simulink model "WaterRunner_closed2"  (R2013a)
settings: Solver=ode23s  StartTime=0.0  StopTime=10  RelTol=1e-3
values from neighbouring files (symbols this model uses):
  Ac = [sum(Ay), sum(Ath), sum(Aph) ... (first row only)    [SimParam_hopper.m]    (also in simParam.m = [2*sum(Ay), 2*sum(Ath))
  dTorqueAmp = 1e-2    (= 0.01)    [SimParam_hopper.m]
  dTorqueFreq = 0.5    [SimParam_hopper.m]    (also in simParam.m = 3.14159265359)
  Filter_Coef = 1000    [SimParam_hopper.m]    (also in simParam.m)
  freq = findSSinput(y,b_water,k_water,A,Fratio,mass*g/4,w0)    [SimParam_hopper.m]    (also in findParams.m = freqs(k); simParam.m; sweepDFomega.m = FREQ(k))
  Gc = [sum(G) - mass*g ; Lx'*G ; Lz'*G]    [SimParam_hopper.m]    (also in simParam.m = [2*sum(G) - mass*g ; Lx'*G ])
  Kdf = 0.25    [SimParam_hopper.m]    (also in simParam.m = 0)
  Ke = diag([0 1])    [simParam.m]
  Mc = [mass 0 0; 0 Ix 0 ; 0 0 Iz]    [SimParam_hopper.m]    (also in simParam.m = [mass 0 ; 0 Ix])
  nullProj = eye(8) - pinvBc*Bc    [SimParam_hopper.m]    (also in simParam.m = eye(4) - pinvBc*Bc)
  omega_0 = freq*ones(8,1)    [SimParam_hopper.m]    (also in findParams.m = freq*ones(4,1); simParam.m = freq*ones(4,1); sweepDFomega.m = freq*ones(4,1))
  pinvBc = pinv(Bc)    [SimParam_hopper.m]    (also in simParam.m)
  tail_density = CF_density    (= 1790)    [simParam.m]
  tail_length = 0.1    [simParam.m]
  theta = 0 *pi/180    (= 0)    [SimParam_hopper.m]    (also in simParam.m)
  y = 0.02    [SimParam_hopper.m]    (also in simParam.m = 0.015)
undefined symbols (not defined in the file or in its folder): X, Y, Z
undefined symbols (not defined in the file): cw_FL_HL, cw_FR_FL, cw_FR_HR, cw_HR_HL, FL_HL_lag, FR_FL_lag, FR_HR_lag, HR_HL_lag, K_d, K_i, K_p, phi0, tail_pad_radius, theta0, water_level, y0
libraries: nesl_utility x38, sm_lib x35, WaterRunner_lib_2 x11, dspstat3 x4, simulink x2
(part 2 of 4)

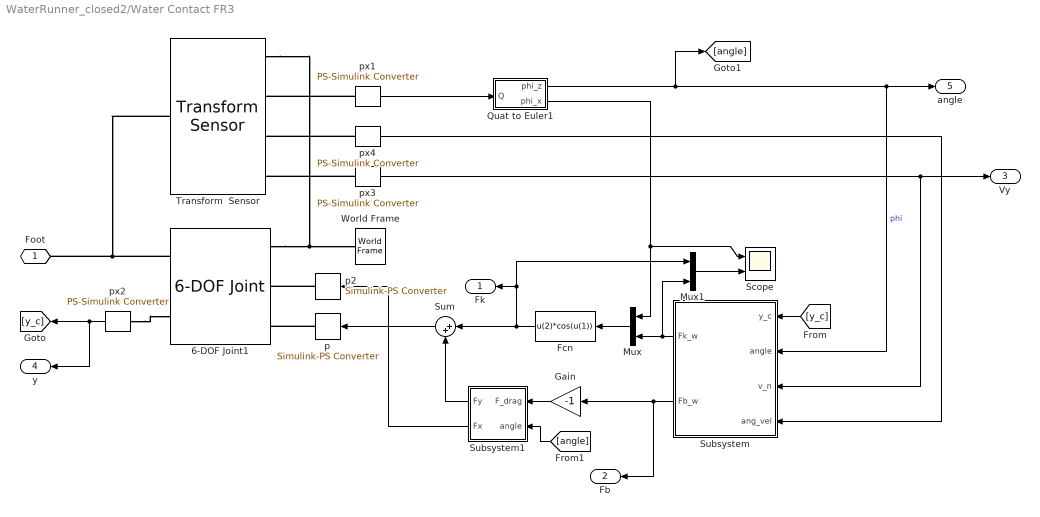
== system WaterRunner_closed2/Water Contact FR3 ==
  6-DOF Joint1 : sm_lib/Joints/6-DOF Joint  SenseConstraintForceX=off  SenseConstraintForceY=off  SenseConstraintForceZ=off  SenseConstraintTorqueX=off  SenseConstraintTorqueY=off  SenseConstraintTorqueZ=off  ConstraintWrenchDir=FollowerOnBase  ConstraintWrenchFrame=BaseFrame  PxEquilibriumPosition=0  PxEquilibriumPositionUnits=m  PxSpringStiffness=0  PxSpringStiffnessUnits=N/m  PxDampingCoefficient=0  PxDampingCoefficientUnits=N/(m/s)  PxActuationMode=TorqueForceActuation  PxSensePosition=off  PxSenseVelocity=off  PxSenseAcceleration=off  PxSenseTorqueForce=off  PxPositionTargetValue=0  PxPositionTargetValueUnits=m  PxPositionTargetSpecify=off  PxPositionTargetPriority=High  PxVelocityTargetValue=0  PxVelocityTargetValueUnits=m/s  PxVelocityTargetSpecify=off  PxVelocityTargetPriority=High  PyEquilibriumPosition=0  PyEquilibriumPositionUnits=m  PySpringStiffness=0  PySpringStiffnessUnits=N/m  PyDampingCoefficient=0  PyDampingCoefficientUnits=N/(m/s)  PyActuationMode=TorqueForceActuation  PySensePosition=on  PySenseVelocity=off  PySenseAcceleration=off  PySenseTorqueForce=off  PyPositionTargetValue=0  PyPositionTargetValueUnits=m  PyPositionTargetSpecify=off  PyPositionTargetPriority=High  PyVelocityTargetValue=0  PyVelocityTargetValueUnits=m/s  PyVelocityTargetSpecify=off  PyVelocityTargetPriority=High  PzEquilibriumPosition=0  PzEquilibriumPositionUnits=m  PzSpringStiffness=0  PzSpringStiffnessUnits=N/m  PzDampingCoefficient=0  PzDampingCoefficientUnits=N/(m/s)  PzActuationMode=NoActuation  PzSensePosition=off  PzSenseVelocity=off  PzSenseAcceleration=off  PzSenseTorqueForce=off  PzPositionTargetValue=0  PzPositionTargetValueUnits=m  PzPositionTargetSpecify=off  PzPositionTargetPriority=High  PzVelocityTargetValue=0  PzVelocityTargetValueUnits=m/s  PzVelocityTargetSpecify=off  PzVelocityTargetPriority=High  SphDefPosRotationMethod=None  SphDefPosRotationAngleUnits=deg  SphDefPosRotationStandardAxis=+Z  SphDefPosRotationAngle=0  SphDefPosRotationArbitraryAxis=[0 0 1]  SphDefPosFollAlignAxisA=+X  SphDefPosBaseAlignAxisA=+Y  SphDefPosFollAlignAxisB=+Y  SphDefPosBaseAlignAxisB=+Z  SphEqPosRotationMethod=None  SphEqPosRotationAngleUnits=deg  SphEqPosRotationStandardAxis=+Z  SphEqPosRotationAngle=0  SphEqPosRotationArbitraryAxis=[0 0 1]  SphEqPosFollAlignAxisA=+X  SphEqPosBaseAlignAxisA=+Y  SphEqPosFollAlignAxisB=+Y  SphEqPosBaseAlignAxisB=+Z  SphSpringStiffness=0  SphSpringStiffnessUnits=N*m/deg  SphDampingCoefficient=0  SphDampingCoefficientUnits=N*m/(deg/s)  SphActuateTorqueX=off  SphActuateTorqueY=off  SphActuateTorqueZ=off  SphActuateTorque=off  SphActuationMode=NoActuation  SphActuationFrame=BaseFrame  SphSensePosition=off  SphSenseVelocityX=off  SphSenseVelocityY=off  SphSenseVelocityZ=off  SphSenseVelocity=off  SphSenseAccelerationX=off  SphSenseAccelerationY=off  SphSenseAccelerationZ=off  SphSenseAcceleration=off  SphSenseTorqueX=off  SphSenseTorqueY=off  SphSenseTorqueZ=off  SphSenseTorqueForce=off  SphSensingFrame=BaseFrame  SphPositionTargetRotationMethod=None  SphPositionTargetRotationAngleUnits=deg  SphPositionTargetRotationStandardAxis=+Z  SphPositionTargetRotationAngle=0  SphPositionTargetRotationArbitraryAxis=[0 0 1]  SphPositionTargetFollAlignAxisA=+X  SphPositionTargetBaseAlignAxisA=+Y  SphPositionTargetFollAlignAxisB=+Y  SphPositionTargetBaseAlignAxisB=+Z  SphPositionTargetSpecify=off  SphPositionTargetPriority=High  SphVelocityTargetValue=[0 0 0]  SphVelocityTargetValueUnits=deg/s  SphVelocityTargetSpecify=off  SphVelocityTargetPriority=High  SphVelocityTargetInFollowerFrame=on  BlockFunction=simmechanics.library.joints.sixdof_joint
  Fcn : Fcn  Expr=u(2)*cos(u(1))
  Gain : Gain  Gain=-1
  Mux : Mux  Inputs=2
  Mux1 : Mux  Inputs=2
  Quat to Euler1 : Subsystem
  Scope : Scope  NumInputPorts=2
      settings: YMin=-0.19~0  YMax=0.04~0.7  SaveName=ScopeData3
  Subsystem : Subsystem
  Subsystem1 : Subsystem
  Sum : Sum  Inputs=|++
  Transform  Sensor : sm_lib/Frames and  Transforms/Transform  Sensor  MeasurementFrame=NonRotatingBase  SenseAngle=off  SenseAxis=off  SenseAngle1=off  SenseAngle2=off  SenseAngle3=off  SenseQ=on  SenseR=off  SenseOmegaX=off  SenseOmegaY=off  SenseOmegaZ=on  SenseOmega1=off  SenseOmega2=off  SenseOmega3=off  SenseQDot=off  SenseRDot=off  SenseAlphaX=off  SenseAlphaY=off  SenseAlphaZ=off  SenseAlpha1=off  SenseAlpha2=off  SenseAlpha3=off  SenseQDDot=off  SenseRDDot=off  SenseX=off  SenseY=off  SenseZ=off  SenseRad=off  SenseAzim=off  SenseDist=off  SenseInc=off  SenseXDot=off  SenseYDot=on  SenseZDot=off  SenseRadDot=off  SenseAzimDot=off  SenseDistDot=off  SenseIncDot=off  SenseXDDot=off  SenseYDDot=off  SenseZDDot=off  SenseRadDDot=off  SenseAzimDDot=off  SenseDistDDot=off  SenseIncDDot=off  BlockFunction=simmechanics.library.frames_transforms.transform_sensor
  World Frame : sm_lib/Frames and  Transforms/World Frame  BlockFunction=simmechanics.library.frames_transforms.world_frame
  p : nesl_utility/Simulink-PS Converter  PhysicalDomain=network_engine_domain  SubClassName=ps_input  LeftPortType=input  RightPortType=output  PseudoPeriodic=off  Frequencies=[]  NoiseDistribution=none  NoiseParameters=[]  Unit=1  AffineConversion=off  InputFiltering=off  SimscapeFilterOrder=1  InputFilterTimeConstant=.001  UdotUserProvided=[]
  p2 : nesl_utility/Simulink-PS Converter  PhysicalDomain=network_engine_domain  SubClassName=ps_input  LeftPortType=input  RightPortType=output  PseudoPeriodic=off  Frequencies=[]  NoiseDistribution=none  NoiseParameters=[]  Unit=1  AffineConversion=off  InputFiltering=off  SimscapeFilterOrder=1  InputFilterTimeConstant=.001  UdotUserProvided=[]
  px{1..4} (4 alike) : nesl_utility/PS-Simulink Converter  PhysicalDomain=network_engine_domain  SubClassName=ps_output  LeftPortType=input  RightPortType=output  PseudoPeriodic=off  Frequencies=[]  Unit=1  AffineConversion=off
  Foot : PMIOPort  Port=1  Side=Left
  Fk : Outport
  Fb : Outport  Port=2
  Vy : Outport  Port=3
  y : Outport  Port=4
  angle : Outport  Port=5
  wires:
  Subsystem/2(Fb_w) -> Gain/1, Fb/1
  px3/1 -> Vy/1, Subsystem/3(v_n)
  Quat to Euler1/1(phi_z) -> [angle], Subsystem/2(angle), angle/1  "phi"
  px1/1 -> Quat to Euler1/1(Q)
  px4/1 -> Subsystem/4(ang_vel)
  px2/1 -> [y_c], y/1
  [y_c] -> Subsystem/1(y_c)
  [angle] -> Subsystem1/2(angle)
  Sum/1 -> p/1
  Subsystem1/1(Fy) -> Sum/2
  Gain/1 -> Subsystem1/1(F_drag)
  Subsystem1/2(Fx) -> p2/1
  Subsystem/1(Fk_w) -> Mux1/2, Mux/2
  Mux/1 -> Fcn/1
  Fcn/1 -> Mux1/1, Fk/1, Sum/1
  Quat to Euler1/2(phi_x) -> Mux/1, Scope/1
  Mux1/1 -> Scope/2
  connections:
  Transform  Sensor/RConn1 -- World Frame/RConn1 -- 6-DOF Joint1/LConn1
  Transform  Sensor/LConn1 -- Foot/RConn1 -- 6-DOF Joint1/RConn1
  px2/LConn1 -- 6-DOF Joint1/RConn2
  p/RConn1 -- 6-DOF Joint1/LConn3
  px1/LConn1 -- Transform  Sensor/RConn2
  p2/RConn1 -- 6-DOF Joint1/LConn2
  px3/LConn1 -- Transform  Sensor/RConn4
  px4/LConn1 -- Transform  Sensor/RConn3

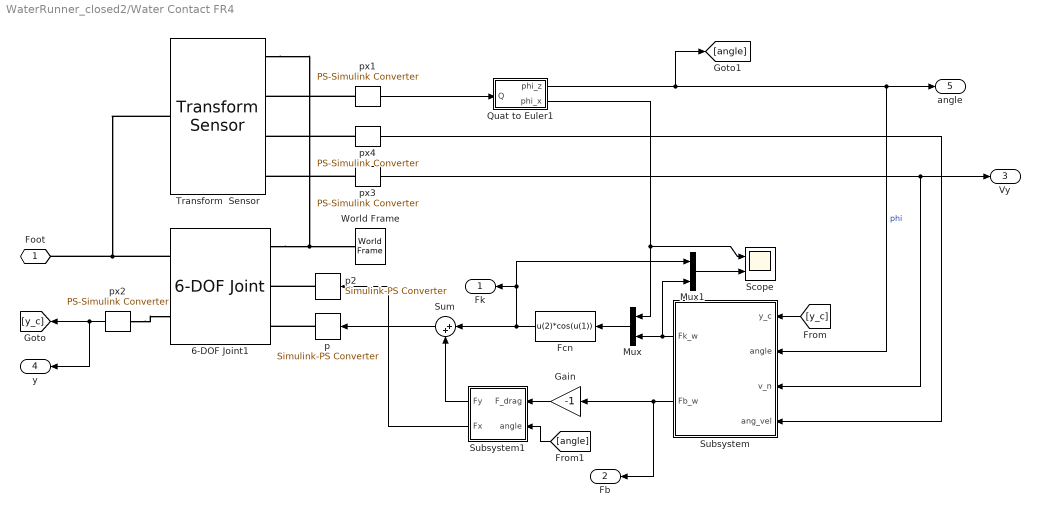
== system WaterRunner_closed2/Water Contact FR4 ==
  6-DOF Joint1 : sm_lib/Joints/6-DOF Joint  SenseConstraintForceX=off  SenseConstraintForceY=off  SenseConstraintForceZ=off  SenseConstraintTorqueX=off  SenseConstraintTorqueY=off  SenseConstraintTorqueZ=off  ConstraintWrenchDir=FollowerOnBase  ConstraintWrenchFrame=BaseFrame  PxEquilibriumPosition=0  PxEquilibriumPositionUnits=m  PxSpringStiffness=0  PxSpringStiffnessUnits=N/m  PxDampingCoefficient=0  PxDampingCoefficientUnits=N/(m/s)  PxActuationMode=TorqueForceActuation  PxSensePosition=off  PxSenseVelocity=off  PxSenseAcceleration=off  PxSenseTorqueForce=off  PxPositionTargetValue=0  PxPositionTargetValueUnits=m  PxPositionTargetSpecify=off  PxPositionTargetPriority=High  PxVelocityTargetValue=0  PxVelocityTargetValueUnits=m/s  PxVelocityTargetSpecify=off  PxVelocityTargetPriority=High  PyEquilibriumPosition=0  PyEquilibriumPositionUnits=m  PySpringStiffness=0  PySpringStiffnessUnits=N/m  PyDampingCoefficient=0  PyDampingCoefficientUnits=N/(m/s)  PyActuationMode=TorqueForceActuation  PySensePosition=on  PySenseVelocity=off  PySenseAcceleration=off  PySenseTorqueForce=off  PyPositionTargetValue=0  PyPositionTargetValueUnits=m  PyPositionTargetSpecify=off  PyPositionTargetPriority=High  PyVelocityTargetValue=0  PyVelocityTargetValueUnits=m/s  PyVelocityTargetSpecify=off  PyVelocityTargetPriority=High  PzEquilibriumPosition=0  PzEquilibriumPositionUnits=m  PzSpringStiffness=0  PzSpringStiffnessUnits=N/m  PzDampingCoefficient=0  PzDampingCoefficientUnits=N/(m/s)  PzActuationMode=NoActuation  PzSensePosition=off  PzSenseVelocity=off  PzSenseAcceleration=off  PzSenseTorqueForce=off  PzPositionTargetValue=0  PzPositionTargetValueUnits=m  PzPositionTargetSpecify=off  PzPositionTargetPriority=High  PzVelocityTargetValue=0  PzVelocityTargetValueUnits=m/s  PzVelocityTargetSpecify=off  PzVelocityTargetPriority=High  SphDefPosRotationMethod=None  SphDefPosRotationAngleUnits=deg  SphDefPosRotationStandardAxis=+Z  SphDefPosRotationAngle=0  SphDefPosRotationArbitraryAxis=[0 0 1]  SphDefPosFollAlignAxisA=+X  SphDefPosBaseAlignAxisA=+Y  SphDefPosFollAlignAxisB=+Y  SphDefPosBaseAlignAxisB=+Z  SphEqPosRotationMethod=None  SphEqPosRotationAngleUnits=deg  SphEqPosRotationStandardAxis=+Z  SphEqPosRotationAngle=0  SphEqPosRotationArbitraryAxis=[0 0 1]  SphEqPosFollAlignAxisA=+X  SphEqPosBaseAlignAxisA=+Y  SphEqPosFollAlignAxisB=+Y  SphEqPosBaseAlignAxisB=+Z  SphSpringStiffness=0  SphSpringStiffnessUnits=N*m/deg  SphDampingCoefficient=0  SphDampingCoefficientUnits=N*m/(deg/s)  SphActuateTorqueX=off  SphActuateTorqueY=off  SphActuateTorqueZ=off  SphActuateTorque=off  SphActuationMode=NoActuation  SphActuationFrame=BaseFrame  SphSensePosition=off  SphSenseVelocityX=off  SphSenseVelocityY=off  SphSenseVelocityZ=off  SphSenseVelocity=off  SphSenseAccelerationX=off  SphSenseAccelerationY=off  SphSenseAccelerationZ=off  SphSenseAcceleration=off  SphSenseTorqueX=off  SphSenseTorqueY=off  SphSenseTorqueZ=off  SphSenseTorqueForce=off  SphSensingFrame=BaseFrame  SphPositionTargetRotationMethod=None  SphPositionTargetRotationAngleUnits=deg  SphPositionTargetRotationStandardAxis=+Z  SphPositionTargetRotationAngle=0  SphPositionTargetRotationArbitraryAxis=[0 0 1]  SphPositionTargetFollAlignAxisA=+X  SphPositionTargetBaseAlignAxisA=+Y  SphPositionTargetFollAlignAxisB=+Y  SphPositionTargetBaseAlignAxisB=+Z  SphPositionTargetSpecify=off  SphPositionTargetPriority=High  SphVelocityTargetValue=[0 0 0]  SphVelocityTargetValueUnits=deg/s  SphVelocityTargetSpecify=off  SphVelocityTargetPriority=High  SphVelocityTargetInFollowerFrame=on  BlockFunction=simmechanics.library.joints.sixdof_joint
  Fcn : Fcn  Expr=u(2)*cos(u(1))
  Gain : Gain  Gain=-1
  Mux : Mux  Inputs=2
  Mux1 : Mux  Inputs=2
  Quat to Euler1 : Subsystem
  Scope : Scope  NumInputPorts=2
      settings: YMin=-0.19~0  YMax=0.04~0.7  SaveName=ScopeData3
  Subsystem : Subsystem
  Subsystem1 : Subsystem
  Sum : Sum  Inputs=|++
  Transform  Sensor : sm_lib/Frames and  Transforms/Transform  Sensor  MeasurementFrame=NonRotatingBase  SenseAngle=off  SenseAxis=off  SenseAngle1=off  SenseAngle2=off  SenseAngle3=off  SenseQ=on  SenseR=off  SenseOmegaX=off  SenseOmegaY=off  SenseOmegaZ=on  SenseOmega1=off  SenseOmega2=off  SenseOmega3=off  SenseQDot=off  SenseRDot=off  SenseAlphaX=off  SenseAlphaY=off  SenseAlphaZ=off  SenseAlpha1=off  SenseAlpha2=off  SenseAlpha3=off  SenseQDDot=off  SenseRDDot=off  SenseX=off  SenseY=off  SenseZ=off  SenseRad=off  SenseAzim=off  SenseDist=off  SenseInc=off  SenseXDot=off  SenseYDot=on  SenseZDot=off  SenseRadDot=off  SenseAzimDot=off  SenseDistDot=off  SenseIncDot=off  SenseXDDot=off  SenseYDDot=off  SenseZDDot=off  SenseRadDDot=off  SenseAzimDDot=off  SenseDistDDot=off  SenseIncDDot=off  BlockFunction=simmechanics.library.frames_transforms.transform_sensor
  World Frame : sm_lib/Frames and  Transforms/World Frame  BlockFunction=simmechanics.library.frames_transforms.world_frame
  p : nesl_utility/Simulink-PS Converter  PhysicalDomain=network_engine_domain  SubClassName=ps_input  LeftPortType=input  RightPortType=output  PseudoPeriodic=off  Frequencies=[]  NoiseDistribution=none  NoiseParameters=[]  Unit=1  AffineConversion=off  InputFiltering=off  SimscapeFilterOrder=1  InputFilterTimeConstant=.001  UdotUserProvided=[]
  p2 : nesl_utility/Simulink-PS Converter  PhysicalDomain=network_engine_domain  SubClassName=ps_input  LeftPortType=input  RightPortType=output  PseudoPeriodic=off  Frequencies=[]  NoiseDistribution=none  NoiseParameters=[]  Unit=1  AffineConversion=off  InputFiltering=off  SimscapeFilterOrder=1  InputFilterTimeConstant=.001  UdotUserProvided=[]
  px{1..4} (4 alike) : nesl_utility/PS-Simulink Converter  PhysicalDomain=network_engine_domain  SubClassName=ps_output  LeftPortType=input  RightPortType=output  PseudoPeriodic=off  Frequencies=[]  Unit=1  AffineConversion=off
  Foot : PMIOPort  Port=1  Side=Left
  Fk : Outport
  Fb : Outport  Port=2
  Vy : Outport  Port=3
  y : Outport  Port=4
  angle : Outport  Port=5
  wires:
  Subsystem/2(Fb_w) -> Gain/1, Fb/1
  px3/1 -> Vy/1, Subsystem/3(v_n)
  Quat to Euler1/1(phi_z) -> [angle], Subsystem/2(angle), angle/1  "phi"
  px1/1 -> Quat to Euler1/1(Q)
  px4/1 -> Subsystem/4(ang_vel)
  px2/1 -> [y_c], y/1
  [y_c] -> Subsystem/1(y_c)
  [angle] -> Subsystem1/2(angle)
  Sum/1 -> p/1
  Subsystem1/1(Fy) -> Sum/2
  Gain/1 -> Subsystem1/1(F_drag)
  Subsystem1/2(Fx) -> p2/1
  Subsystem/1(Fk_w) -> Mux1/2, Mux/2
  Mux/1 -> Fcn/1
  Fcn/1 -> Mux1/1, Fk/1, Sum/1
  Quat to Euler1/2(phi_x) -> Mux/1, Scope/1
  Mux1/1 -> Scope/2
  connections:
  Transform  Sensor/RConn1 -- World Frame/RConn1 -- 6-DOF Joint1/LConn1
  Transform  Sensor/LConn1 -- Foot/RConn1 -- 6-DOF Joint1/RConn1
  px2/LConn1 -- 6-DOF Joint1/RConn2
  p/RConn1 -- 6-DOF Joint1/LConn3
  px1/LConn1 -- Transform  Sensor/RConn2
  p2/RConn1 -- 6-DOF Joint1/LConn2
  px3/LConn1 -- Transform  Sensor/RConn4
  px4/LConn1 -- Transform  Sensor/RConn3

== system WaterRunner_closed2/desired output ==
  Mux1 : Mux  Inputs=2
  m : Constant  Value=y
  m1 : Constant  Value=theta
  desired output : Outport
  wires:
  m/1 -> Mux1/1  "height"
  Mux1/1 -> desired output/1
  m1/1 -> Mux1/2

== system WaterRunner_closed2/observer ==
  Gain : Gain  Gain=-1
  Gain1 : Gain  Gain=-1
  Integrator : Integrator
  Integrator1 : Integrator
  Mux{,1..2,5} (4 alike) : Mux  Inputs=2
  PS-Simulink Converter{,1..5} (6 alike) : nesl_utility/PS-Simulink Converter  PhysicalDomain=network_engine_domain  SubClassName=ps_output  LeftPortType=input  RightPortType=output  PseudoPeriodic=off  Frequencies=[]  Unit=1  AffineConversion=off
  Transform  Sensor : sm_lib/Frames and  Transforms/Transform  Sensor  MeasurementFrame=World  SenseAngle=off  SenseAxis=off  SenseAngle1=off  SenseAngle2=off  SenseAngle3=off  SenseQ=off  SenseR=off  SenseOmegaX=on  SenseOmegaY=off  SenseOmegaZ=on  SenseOmega1=off  SenseOmega2=off  SenseOmega3=off  SenseQDot=off  SenseRDot=off  SenseAlphaX=on  SenseAlphaY=off  SenseAlphaZ=on  SenseAlpha1=off  SenseAlpha2=off  SenseAlpha3=off  SenseQDDot=off  SenseRDDot=off  SenseX=off  SenseY=on  SenseZ=off  SenseRad=off  SenseAzim=off  SenseDist=off  SenseInc=off  SenseXDot=off  SenseYDot=off  SenseZDot=off  SenseRadDot=off  SenseAzimDot=off  SenseDistDot=off  SenseIncDot=off  SenseXDDot=off  SenseYDDot=on  SenseZDDot=off  SenseRadDDot=off  SenseAzimDDot=off  SenseDistDDot=off  SenseIncDDot=off  BlockFunction=simmechanics.library.frames_transforms.transform_sensor
  averaging1 : Subsystem  mask{T_win=2*pi/freq, x_init=y0}
      mask prompts: T_win "window (s)"; x_init "Initial condition"
  averaging2 : Subsystem  mask{T_win=2*pi/freq, x_init=0}
      mask prompts: T_win "window (s)"; x_init "Initial condition"
  averaging3 : Subsystem  mask{T_win=2*pi/freq, x_init=[0 0]}
      mask prompts: T_win "window (s)"; x_init "Initial condition"
  averaging5 : Subsystem  mask{T_win=2*pi/freq, x_init=[theta0 phi0]}
      mask prompts: T_win "window (s)"; x_init "Initial condition"
  Base : PMIOPort  Port=1  Side=Left
  Follower : PMIOPort  Port=2  Side=Left
  output : Outport
  accel : Outport  Port=2
  wires:
  Mux5/1 -> output/1
  Mux/1 -> averaging5/1(in)
  PS-Simulink Converter/1 -> Integrator/1
  Integrator1/1 -> Mux/2
  Integrator/1 -> Gain/1
  PS-Simulink Converter1/1 -> Integrator1/1
  PS-Simulink Converter2/1 -> averaging1/1(in)
  averaging1/1(out) -> Mux5/1
  Mux2/1 -> accel/1
  Mux1/1 -> averaging3/1(in)
  PS-Simulink Converter4/1 -> Mux1/2
  PS-Simulink Converter3/1 -> Gain1/1
  PS-Simulink Converter5/1 -> averaging2/1(in)
  averaging2/1(out) -> Mux2/1
  averaging5/1(out) -> Mux5/2
  averaging3/1(out) -> Mux2/2
  Gain/1 -> Mux/1
  Gain1/1 -> Mux1/1
  connections:
  Transform  Sensor/LConn1 -- Base/RConn1
  PS-Simulink Converter/LConn1 -- Transform  Sensor/RConn2
  Follower/RConn1 -- Transform  Sensor/RConn1
  PS-Simulink Converter1/LConn1 -- Transform  Sensor/RConn3
  PS-Simulink Converter2/LConn1 -- Transform  Sensor/RConn6
  PS-Simulink Converter3/LConn1 -- Transform  Sensor/RConn4
  PS-Simulink Converter4/LConn1 -- Transform  Sensor/RConn5
  PS-Simulink Converter5/LConn1 -- Transform  Sensor/RConn7

== system WaterRunner_closed2/CPG_Network/FL_HL lag ==
  In1 : Inport
  In2 : Inport  Port=2
  Constant : Constant  Value=d_phase
  Gain : Gain  Gain=-1
  Sum : Sum  Inputs=--+
  sin : Fcn  Expr=coupling_weight*sin(u(1))
  Out1 : Outport
  Out2 : Outport  Port=2
  wires:
  Sum/1 -> sin/1
  sin/1 -> Gain/1, Out1/1
  Constant/1 -> Sum/2
  In1/1 -> Sum/1
  In2/1 -> Sum/3
  Gain/1 -> Out2/1

== system WaterRunner_closed2/CPG_Network/FR_FL lag ==
  In1 : Inport
  In2 : Inport  Port=2
  Constant : Constant  Value=d_phase
  Gain : Gain  Gain=-1
  Sum : Sum  Inputs=--+
  sin : Fcn  Expr=coupling_weight*sin(u(1))
  Out1 : Outport
  Out2 : Outport  Port=2
  wires:
  Sum/1 -> sin/1
  sin/1 -> Gain/1, Out1/1
  Constant/1 -> Sum/2
  In1/1 -> Sum/1
  In2/1 -> Sum/3
  Gain/1 -> Out2/1

== system WaterRunner_closed2/CPG_Network/FR_HR lag ==
  In1 : Inport
  In2 : Inport  Port=2
  Constant : Constant  Value=d_phase
  Gain : Gain  Gain=-1
  Sum : Sum  Inputs=--+
  sin : Fcn  Expr=coupling_weight*sin(u(1))
  Out1 : Outport
  Out2 : Outport  Port=2
  wires:
  Gain/1 -> Out2/1
  In2/1 -> Sum/3
  In1/1 -> Sum/1
  Constant/1 -> Sum/2
  sin/1 -> Out1/1, Gain/1
  Sum/1 -> sin/1

== system WaterRunner_closed2/CPG_Network/Front_Left ==
  force : Inport
  Constant3 : Constant  Value=freq
  Integrator3 : Integrator  InitialCondition=init_phi + 0.001*rand
  Mod 2pi : Fcn  Expr=atan2(sin(u(1)-pi),cos(u(1)-pi))+pi
  Sum2 : Sum  Inputs=|++
  vel : Outport
  phase : Outport  Port=2
  wires:
  force/1 -> Sum2/2
  Sum2/1 -> vel/1, Integrator3/1
  Constant3/1 -> Sum2/1
  Integrator3/1 -> Mod 2pi/1
  Mod 2pi/1 -> phase/1

== system WaterRunner_closed2/CPG_Network/Front_Right ==
  force : Inport
  Constant3 : Constant  Value=freq
  Integrator3 : Integrator  InitialCondition=init_phi + 0.001*rand
  Mod 2pi : Fcn  Expr=atan2(sin(u(1)-pi),cos(u(1)-pi))+pi
  Sum2 : Sum  Inputs=|++
  vel : Outport
  phase : Outport  Port=2
  wires:
  Mod 2pi/1 -> phase/1
  Integrator3/1 -> Mod 2pi/1
  Constant3/1 -> Sum2/1
  Sum2/1 -> Integrator3/1, vel/1
  force/1 -> Sum2/2

== system WaterRunner_closed2/CPG_Network/HR_HL lag ==
  In1 : Inport
  In2 : Inport  Port=2
  Constant : Constant  Value=d_phase
  Gain : Gain  Gain=-1
  Sum : Sum  Inputs=--+
  sin : Fcn  Expr=coupling_weight*sin(u(1))
  Out1 : Outport
  Out2 : Outport  Port=2
  wires:
  Gain/1 -> Out2/1
  In2/1 -> Sum/3
  In1/1 -> Sum/1
  Constant/1 -> Sum/2
  sin/1 -> Out1/1, Gain/1
  Sum/1 -> sin/1

== system WaterRunner_closed2/CPG_Network/Hind_Left ==
  force : Inport
  Constant3 : Constant  Value=freq
  Integrator3 : Integrator  InitialCondition=init_phi + 0.001*rand
  Mod 2pi : Fcn  Expr=atan2(sin(u(1)-pi),cos(u(1)-pi))+pi
  Sum2 : Sum  Inputs=|++
  vel : Outport
  phase : Outport  Port=2
  wires:
  force/1 -> Sum2/2
  Sum2/1 -> vel/1, Integrator3/1
  Constant3/1 -> Sum2/1
  Integrator3/1 -> Mod 2pi/1
  Mod 2pi/1 -> phase/1

== system WaterRunner_closed2/CPG_Network/Hind_Right ==
  force : Inport
  Constant3 : Constant  Value=freq
  Integrator3 : Integrator  InitialCondition=init_phi + 0.001*rand
  Mod 2pi : Fcn  Expr=atan2(sin(u(1)-pi),cos(u(1)-pi))+pi
  Sum2 : Sum  Inputs=|++
  vel : Outport
  phase : Outport  Port=2
  wires:
  force/1 -> Sum2/2
  Sum2/1 -> vel/1, Integrator3/1
  Constant3/1 -> Sum2/1
  Integrator3/1 -> Mod 2pi/1
  Mod 2pi/1 -> phase/1

== system WaterRunner_closed2/CPG_Network/split FL ==
  w_pos : Inport
  phase : Inport  Port=2
  w_neg : Inport  Port=3
  Product : Product  RndMeth=Zero
  Product1 : Product  RndMeth=Zero
  Sum2 : Sum  Inputs=|++
  enable : Subsystem
  Force : Outport
  wires:
  Product/1 -> Sum2/1
  w_pos/1 -> Product/1
  w_neg/1 -> Product1/1
  Product1/1 -> Sum2/2
  enable/1(pos) -> Product/2
  enable/2(neg) -> Product1/2
  Sum2/1 -> Force/1
  phase/1 -> enable/1(in)

== system WaterRunner_closed2/CPG_Network/split FL1 ==
  w_pos : Inport
  phase : Inport  Port=2
  w_neg : Inport  Port=3
  Product : Product  RndMeth=Zero
  Product1 : Product  RndMeth=Zero
  Sum2 : Sum  Inputs=|++
  enable : Subsystem
  Force : Outport
  wires:
  Product/1 -> Sum2/1
  w_pos/1 -> Product/1
  w_neg/1 -> Product1/1
  Product1/1 -> Sum2/2
  enable/1(pos) -> Product/2
  enable/2(neg) -> Product1/2
  Sum2/1 -> Force/1
  phase/1 -> enable/1(in)

== system WaterRunner_closed2/CPG_Network/split FL2 ==
  w_pos : Inport
  phase : Inport  Port=2
  w_neg : Inport  Port=3
  Product : Product  RndMeth=Zero
  Product1 : Product  RndMeth=Zero
  Sum2 : Sum  Inputs=|++
  enable : Subsystem
  Force : Outport
  wires:
  phase/1 -> enable/1(in)
  Sum2/1 -> Force/1
  enable/2(neg) -> Product1/2
  enable/1(pos) -> Product/2
  Product1/1 -> Sum2/2
  w_neg/1 -> Product1/1
  w_pos/1 -> Product/1
  Product/1 -> Sum2/1

== system WaterRunner_closed2/CPG_Network/split FL3 ==
  w_pos : Inport
  phase : Inport  Port=2
  w_neg : Inport  Port=3
  Product : Product  RndMeth=Zero
  Product1 : Product  RndMeth=Zero
  Sum2 : Sum  Inputs=|++
  enable : Subsystem
  Force : Outport
  wires:
  Product/1 -> Sum2/1
  w_pos/1 -> Product/1
  w_neg/1 -> Product1/1
  Product1/1 -> Sum2/2
  enable/1(pos) -> Product/2
  enable/2(neg) -> Product1/2
  Sum2/1 -> Force/1
  phase/1 -> enable/1(in)

== system WaterRunner_closed2/Controller/PID ==
  anti windup : Inport
  err_x : Inport  Port=2
  Derivative Gain : Gain  Gain=D  Multiplication=Matrix(K*u)
  Gain : Gain  Gain=Filter_Coef
  Integral Gain : Gain  DisableCoverage=on  Gain=I  Multiplication=Matrix(K*u)
  Integrator : Integrator
  Integrator1 : Integrator
  Proportional Gain : Gain  Gain=P  Multiplication=Matrix(K*u)
  Sum : Sum  Inputs=|+-
  Sum1 : Sum  Inputs=++|
  Sum11 : Sum  Inputs=+++
  Out1 : Outport
  wires:
  Proportional Gain/1 -> Sum11/1
  Sum11/1 -> Out1/1
  Integrator/1 -> Sum11/2
  Gain/1 -> Integrator1/1, Sum11/3
  err_x/1 -> Derivative Gain/1, Integral Gain/1, Proportional Gain/1
  Derivative Gain/1 -> Sum/1
  Sum/1 -> Gain/1
  Integrator1/1 -> Sum/2
  Integral Gain/1 -> Sum1/2
  Sum1/1 -> Integrator/1
  anti windup/1 -> Sum1/1

== system WaterRunner_closed2/Controller/Prefer Duty Factor ==
  omega : Inport
  Demux1 : Demux
  Mean4 : dspstat3/Mean  run=off  reset_popup=None  InputProcessing=Columns as channels (frame based)  directionMode=Each column  dimension=1  treatSBRowAsCol=on  roiEnable=off  roiType=Rectangles  roiPortion=Entire ROI  roiOutput=Individual statistics for each ROI  roiFlag=off  outputDataTypeStr=Inherit: Same as accumulator  outputLastDataTypeStr=Inherit: Same as accumulator  outputMin=[]  outputMax=[]  roundingMode=Floor  overflowMode=off
  Mean5 : dspstat3/Mean  run=off  reset_popup=None  InputProcessing=Columns as channels (frame based)  directionMode=Each column  dimension=1  treatSBRowAsCol=on  roiEnable=off  roiType=Rectangles  roiPortion=Entire ROI  roiOutput=Individual statistics for each ROI  roiFlag=off  outputDataTypeStr=Inherit: Same as accumulator  outputLastDataTypeStr=Inherit: Same as accumulator  outputMin=[]  outputMax=[]  roundingMode=Floor  overflowMode=off
  Mux1 : Mux
  Mux6 : Mux  Inputs=2
  Mux7 : Mux  Inputs=2
  omega _0 : Outport
  wires:
  Mean5/1 -> Mux1/3, Mux1/4
  Demux1/4 -> Mux7/2
  Demux1/3 -> Mux7/1
  Demux1/2 -> Mux6/2
  Mux6/1 -> Mean4/1
  Mux7/1 -> Mean5/1
  omega/1 -> Demux1/1
  Demux1/1 -> Mux6/1
  Mux1/1 -> omega _0/1
  Mean4/1 -> Mux1/1, Mux1/2

== system WaterRunner_closed2/Controller/Prefer No Duty Factor ==
  omega : Inport
  Demux1 : Demux
  Mean1 : dspstat3/Mean  run=off  reset_popup=None  InputProcessing=Columns as channels (frame based)  directionMode=Each column  dimension=1  treatSBRowAsCol=on  roiEnable=off  roiType=Rectangles  roiPortion=Entire ROI  roiOutput=Individual statistics for each ROI  roiFlag=off  outputDataTypeStr=Inherit: Same as accumulator  outputLastDataTypeStr=Inherit: Same as accumulator  outputMin=[]  outputMax=[]  roundingMode=Floor  overflowMode=off
  Mean2 : dspstat3/Mean  run=off  reset_popup=None  InputProcessing=Columns as channels (frame based)  directionMode=Each column  dimension=1  treatSBRowAsCol=on  roiEnable=off  roiType=Rectangles  roiPortion=Entire ROI  roiOutput=Individual statistics for each ROI  roiFlag=off  outputDataTypeStr=Inherit: Same as accumulator  outputLastDataTypeStr=Inherit: Same as accumulator  outputMin=[]  outputMax=[]  roundingMode=Floor  overflowMode=off
  Mux1 : Mux
  Mux2 : Mux  Inputs=2
  Mux3 : Mux  Inputs=2
  omega_0 : Outport
  wires:
  Demux1/4 -> Mux3/2
  Demux1/3 -> Mux2/2
  Mean2/1 -> Mux1/4, Mux1/2
  omega/1 -> Demux1/1
  Mean1/1 -> Mux1/1, Mux1/3
  Mux1/1 -> omega_0/1
  Demux1/2 -> Mux3/1
  Mux3/1 -> Mean2/1
  Mux2/1 -> Mean1/1
  Demux1/1 -> Mux2/1

== system WaterRunner_closed2/Tail/Water Contact HR1 ==
  6-DOF Joint2 : sm_lib/Joints/6-DOF Joint  SenseConstraintForceX=off  SenseConstraintForceY=off  SenseConstraintForceZ=off  SenseConstraintTorqueX=off  SenseConstraintTorqueY=off  SenseConstraintTorqueZ=off  ConstraintWrenchDir=FollowerOnBase  ConstraintWrenchFrame=BaseFrame  PxEquilibriumPosition=0  PxEquilibriumPositionUnits=m  PxSpringStiffness=0  PxSpringStiffnessUnits=N/m  PxDampingCoefficient=0  PxDampingCoefficientUnits=N/(m/s)  PxActuationMode=TorqueForceActuation  PxSensePosition=off  PxSenseVelocity=off  PxSenseAcceleration=off  PxSenseTorqueForce=off  PxPositionTargetValue=0  PxPositionTargetValueUnits=m  PxPositionTargetSpecify=off  PxPositionTargetPriority=High  PxVelocityTargetValue=0  PxVelocityTargetValueUnits=m/s  PxVelocityTargetSpecify=off  PxVelocityTargetPriority=High  PyEquilibriumPosition=0  PyEquilibriumPositionUnits=m  PySpringStiffness=0  PySpringStiffnessUnits=N/m  PyDampingCoefficient=0  PyDampingCoefficientUnits=N/(m/s)  PyActuationMode=TorqueForceActuation  PySensePosition=on  PySenseVelocity=off  PySenseAcceleration=off  PySenseTorqueForce=off  PyPositionTargetValue=0  PyPositionTargetValueUnits=m  PyPositionTargetSpecify=off  PyPositionTargetPriority=High  PyVelocityTargetValue=0  PyVelocityTargetValueUnits=m/s  PyVelocityTargetSpecify=off  PyVelocityTargetPriority=High  PzEquilibriumPosition=0  PzEquilibriumPositionUnits=m  PzSpringStiffness=0  PzSpringStiffnessUnits=N/m  PzDampingCoefficient=0  PzDampingCoefficientUnits=N/(m/s)  PzActuationMode=NoActuation  PzSensePosition=off  PzSenseVelocity=off  PzSenseAcceleration=off  PzSenseTorqueForce=off  PzPositionTargetValue=0  PzPositionTargetValueUnits=m  PzPositionTargetSpecify=off  PzPositionTargetPriority=High  PzVelocityTargetValue=0  PzVelocityTargetValueUnits=m/s  PzVelocityTargetSpecify=off  PzVelocityTargetPriority=High  SphDefPosRotationMethod=None  SphDefPosRotationAngleUnits=deg  SphDefPosRotationStandardAxis=+Z  SphDefPosRotationAngle=0  SphDefPosRotationArbitraryAxis=[0 0 1]  SphDefPosFollAlignAxisA=+X  SphDefPosBaseAlignAxisA=+Y  SphDefPosFollAlignAxisB=+Y  SphDefPosBaseAlignAxisB=+Z  SphEqPosRotationMethod=None  SphEqPosRotationAngleUnits=deg  SphEqPosRotationStandardAxis=+Z  SphEqPosRotationAngle=0  SphEqPosRotationArbitraryAxis=[0 0 1]  SphEqPosFollAlignAxisA=+X  SphEqPosBaseAlignAxisA=+Y  SphEqPosFollAlignAxisB=+Y  SphEqPosBaseAlignAxisB=+Z  SphSpringStiffness=0  SphSpringStiffnessUnits=N*m/deg  SphDampingCoefficient=0  SphDampingCoefficientUnits=N*m/(deg/s)  SphActuateTorqueX=off  SphActuateTorqueY=off  SphActuateTorqueZ=off  SphActuateTorque=off  SphActuationMode=NoActuation  SphActuationFrame=BaseFrame  SphSensePosition=off  SphSenseVelocityX=off  SphSenseVelocityY=off  SphSenseVelocityZ=off  SphSenseVelocity=off  SphSenseAccelerationX=off  SphSenseAccelerationY=off  SphSenseAccelerationZ=off  SphSenseAcceleration=off  SphSenseTorqueX=off  SphSenseTorqueY=off  SphSenseTorqueZ=off  SphSenseTorqueForce=off  SphSensingFrame=BaseFrame  SphPositionTargetRotationMethod=None  SphPositionTargetRotationAngleUnits=deg  SphPositionTargetRotationStandardAxis=+Z  SphPositionTargetRotationAngle=0  SphPositionTargetRotationArbitraryAxis=[0 0 1]  SphPositionTargetFollAlignAxisA=+X  SphPositionTargetBaseAlignAxisA=+Y  SphPositionTargetFollAlignAxisB=+Y  SphPositionTargetBaseAlignAxisB=+Z  SphPositionTargetSpecify=off  SphPositionTargetPriority=High  SphVelocityTargetValue=[0 0 0]  SphVelocityTargetValueUnits=deg/s  SphVelocityTargetSpecify=off  SphVelocityTargetPriority=High  SphVelocityTargetInFollowerFrame=on  BlockFunction=simmechanics.library.joints.sixdof_joint
  Gain : Gain  Gain=-1
  Gain1 : Gain  Gain=-1
  Quat to Euler1 : WaterRunner_lib_2/Water Contact FR/Quat to Euler1
  Subsystem1 : WaterRunner_lib_2/Water Contact FR/Subsystem1
  Transform  Sensor : sm_lib/Frames and  Transforms/Transform  Sensor  MeasurementFrame=NonRotatingBase  SenseAngle=off  SenseAxis=off  SenseAngle1=off  SenseAngle2=off  SenseAngle3=off  SenseQ=on  SenseR=off  SenseOmegaX=off  SenseOmegaY=off  SenseOmegaZ=on  SenseOmega1=off  SenseOmega2=off  SenseOmega3=off  SenseQDot=off  SenseRDot=off  SenseAlphaX=off  SenseAlphaY=off  SenseAlphaZ=off  SenseAlpha1=off  SenseAlpha2=off  SenseAlpha3=off  SenseQDDot=off  SenseRDDot=off  SenseX=off  SenseY=off  SenseZ=off  SenseRad=off  SenseAzim=off  SenseDist=off  SenseInc=off  SenseXDot=off  SenseYDot=on  SenseZDot=off  SenseRadDot=off  SenseAzimDot=off  SenseDistDot=off  SenseIncDot=off  SenseXDDot=off  SenseYDDot=off  SenseZDDot=off  SenseRadDDot=off  SenseAzimDDot=off  SenseDistDDot=off  SenseIncDDot=off  BlockFunction=simmechanics.library.frames_transforms.transform_sensor
  World Frame1 : sm_lib/Frames and  Transforms/World Frame  BlockFunction=simmechanics.library.frames_transforms.world_frame
  p : nesl_utility/Simulink-PS Converter  PhysicalDomain=network_engine_domain  SubClassName=ps_input  LeftPortType=input  RightPortType=output  PseudoPeriodic=off  Frequencies=[]  NoiseDistribution=none  NoiseParameters=[]  Unit=1  AffineConversion=off  InputFiltering=off  SimscapeFilterOrder=1  InputFilterTimeConstant=.001  UdotUserProvided=[]
  p2 : nesl_utility/Simulink-PS Converter  PhysicalDomain=network_engine_domain  SubClassName=ps_input  LeftPortType=input  RightPortType=output  PseudoPeriodic=off  Frequencies=[]  NoiseDistribution=none  NoiseParameters=[]  Unit=1  AffineConversion=off  InputFiltering=off  SimscapeFilterOrder=1  InputFilterTimeConstant=.001  UdotUserProvided=[]
  px{1..4} (4 alike) : nesl_utility/PS-Simulink Converter  PhysicalDomain=network_engine_domain  SubClassName=ps_output  LeftPortType=input  RightPortType=output  PseudoPeriodic=off  Frequencies=[]  Unit=1  AffineConversion=off
  water_model : Subsystem  mask{Cd=0.703, density=1000, y_w=water_level, R=tail_pad_radius, g=-9.81}
      mask prompts: Cd "Drag Coefficient"; y_w "Water level"; R "Foot Radius"; g "Gravity constant (use negative)"
  Foot : PMIOPort  Port=1  Side=Left
  Fb : Outport
  wires:
  water_model/1(Fb_w) -> Fb/1, Gain/1
  px3/1 -> water_model/3(v_n)
  Quat to Euler1/1 -> [angle], water_model/2(angle)  "phi"
  px1/1 -> Quat to Euler1/1
  px4/1 -> water_model/4(ang_vel)
  px2/1 -> [y_c]
  [y_c] -> water_model/1(y_c)
  [angle] -> Subsystem1/2
  Subsystem1/2 -> Gain1/1
  Subsystem1/1 -> p/1
  Gain/1 -> Subsystem1/1
  Gain1/1 -> p2/1
  connections:
  World Frame1/RConn1 -- Transform  Sensor/RConn1 -- 6-DOF Joint2/LConn1
  Transform  Sensor/LConn1 -- Foot/RConn1 -- 6-DOF Joint2/RConn1
  Transform  Sensor/RConn4 -- px3/LConn1
  px4/LConn1 -- Transform  Sensor/RConn3
  p2/RConn1 -- 6-DOF Joint2/LConn2
  p/RConn1 -- 6-DOF Joint2/LConn3
  px2/LConn1 -- 6-DOF Joint2/RConn2
  px1/LConn1 -- Transform  Sensor/RConn2

== system WaterRunner_closed2/Water Contact FR1/Quat to Euler1 ==
  Q : Inport
  f1 : Fcn  Expr=atan2( 2*(u(1)*u(2) + u(3)*u(4)) , 1-2*(u(2)^2+u(3)^2) )
  f3 : Fcn  Expr=atan2( 2*(u(1)*u(4) + u(2)*u(3)) , 1-2*(u(3)^2+u(4)^2) )
  phi_z : Outport
  phi_x : Outport  Port=2
  wires:
  Q/1 -> f1/1, f3/1
  f3/1 -> phi_z/1
  f1/1 -> phi_x/1

== system WaterRunner_closed2/Water Contact FR1/Subsystem ==
  y_c : Inport
  angle : Inport  Port=2
  v_n : Inport  Port=3
  ang_vel : Inport  Port=4
  Switch : Switch
  Switch1 : Switch
  water_model : Subsystem  mask{Cd=0.703, density=1000, y_w=water_level, R=0.02, g=-9.81}
      mask prompts: Cd "Drag Coefficient"; y_w "Water level"; R "Foot Radius"; g "Gravity constant (use negative)"
  water_model1 : Subsystem  mask{Cd=0.703, density=1000, y_w=water_level, R=0.005, g=-9.81}
      mask prompts: Cd "Drag Coefficient"; y_w "Water level"; R "Foot Radius"; g "Gravity constant (use negative)"
  Fk_w : Outport
  Fb_w : Outport  Port=2
  wires:
  angle/1 -> water_model1/2(angle), water_model/2(angle)
  ang_vel/1 -> water_model1/4(ang_vel), water_model/4(ang_vel)
  y_c/1 -> water_model1/1(y_c), water_model/1(y_c)
  v_n/1 -> water_model1/3(v_n), Switch/2, Switch1/2, water_model/3(v_n)
  water_model/1(Fk_w) -> Switch/1
  water_model/2(Fb_w) -> Switch1/1
  Switch/1 -> Fk_w/1
  water_model1/1(Fk_w) -> Switch/3
  water_model1/2(Fb_w) -> Switch1/3
  Switch1/1 -> Fb_w/1

== system WaterRunner_closed2/Water Contact FR1/Subsystem1 ==
  F_drag : Inport
  angle : Inport  Port=2
  Mux : Mux  Inputs=2
  fcosq : Fcn  Expr=u(1)*cos(u(2))
  fsinq : Fcn  Expr=u(1)*sin(u(2))
  Fy : Outport
  Fx : Outport  Port=2
  wires:
  angle/1 -> Mux/2
  fcosq/1 -> Fy/1
  F_drag/1 -> Mux/1
  Mux/1 -> fcosq/1, fsinq/1
  fsinq/1 -> Fx/1

== system WaterRunner_closed2/Water Contact FR2/Quat to Euler1 ==
  Q : Inport
  f1 : Fcn  Expr=atan2( 2*(u(1)*u(2) + u(3)*u(4)) , 1-2*(u(2)^2+u(3)^2) )
  f3 : Fcn  Expr=atan2( 2*(u(1)*u(4) + u(2)*u(3)) , 1-2*(u(3)^2+u(4)^2) )
  phi_z : Outport
  phi_x : Outport  Port=2
  wires:
  Q/1 -> f1/1, f3/1
  f3/1 -> phi_z/1
  f1/1 -> phi_x/1

== system WaterRunner_closed2/Water Contact FR2/Subsystem ==
  y_c : Inport
  angle : Inport  Port=2
  v_n : Inport  Port=3
  ang_vel : Inport  Port=4
  Switch : Switch
  Switch1 : Switch
  water_model : Subsystem  mask{Cd=0.703, density=1000, y_w=water_level, R=0.02, g=-9.81}
      mask prompts: Cd "Drag Coefficient"; y_w "Water level"; R "Foot Radius"; g "Gravity constant (use negative)"
  water_model1 : Subsystem  mask{Cd=0.703, density=1000, y_w=water_level, R=0.005, g=-9.81}
      mask prompts: Cd "Drag Coefficient"; y_w "Water level"; R "Foot Radius"; g "Gravity constant (use negative)"
  Fk_w : Outport
  Fb_w : Outport  Port=2
  wires:
  angle/1 -> water_model1/2(angle), water_model/2(angle)
  ang_vel/1 -> water_model1/4(ang_vel), water_model/4(ang_vel)
  y_c/1 -> water_model1/1(y_c), water_model/1(y_c)
  v_n/1 -> water_model1/3(v_n), Switch/2, Switch1/2, water_model/3(v_n)
  water_model/1(Fk_w) -> Switch/1
  water_model/2(Fb_w) -> Switch1/1
  Switch/1 -> Fk_w/1
  water_model1/1(Fk_w) -> Switch/3
  water_model1/2(Fb_w) -> Switch1/3
  Switch1/1 -> Fb_w/1

== system WaterRunner_closed2/Water Contact FR2/Subsystem1 ==
  F_drag : Inport
  angle : Inport  Port=2
  Mux : Mux  Inputs=2
  fcosq : Fcn  Expr=u(1)*cos(u(2))
  fsinq : Fcn  Expr=u(1)*sin(u(2))
  Fy : Outport
  Fx : Outport  Port=2
  wires:
  angle/1 -> Mux/2
  fcosq/1 -> Fy/1
  F_drag/1 -> Mux/1
  Mux/1 -> fcosq/1, fsinq/1
  fsinq/1 -> Fx/1

== system WaterRunner_closed2/Water Contact FR3/Quat to Euler1 ==
  Q : Inport
  f1 : Fcn  Expr=atan2( 2*(u(1)*u(2) + u(3)*u(4)) , 1-2*(u(2)^2+u(3)^2) )
  f3 : Fcn  Expr=atan2( 2*(u(1)*u(4) + u(2)*u(3)) , 1-2*(u(3)^2+u(4)^2) )
  phi_z : Outport
  phi_x : Outport  Port=2
  wires:
  Q/1 -> f1/1, f3/1
  f3/1 -> phi_z/1
  f1/1 -> phi_x/1

== system WaterRunner_closed2/Water Contact FR3/Subsystem ==
  y_c : Inport
  angle : Inport  Port=2
  v_n : Inport  Port=3
  ang_vel : Inport  Port=4
  Switch : Switch
  Switch1 : Switch
  water_model : Subsystem  mask{Cd=0.703, density=1000, y_w=water_level, R=0.02, g=-9.81}
      mask prompts: Cd "Drag Coefficient"; y_w "Water level"; R "Foot Radius"; g "Gravity constant (use negative)"
  water_model1 : Subsystem  mask{Cd=0.703, density=1000, y_w=water_level, R=0.005, g=-9.81}
      mask prompts: Cd "Drag Coefficient"; y_w "Water level"; R "Foot Radius"; g "Gravity constant (use negative)"
  Fk_w : Outport
  Fb_w : Outport  Port=2
  wires:
  angle/1 -> water_model1/2(angle), water_model/2(angle)
  ang_vel/1 -> water_model1/4(ang_vel), water_model/4(ang_vel)
  y_c/1 -> water_model1/1(y_c), water_model/1(y_c)
  v_n/1 -> water_model1/3(v_n), Switch/2, Switch1/2, water_model/3(v_n)
  water_model/1(Fk_w) -> Switch/1
  water_model/2(Fb_w) -> Switch1/1
  Switch/1 -> Fk_w/1
  water_model1/1(Fk_w) -> Switch/3
  water_model1/2(Fb_w) -> Switch1/3
  Switch1/1 -> Fb_w/1

== system WaterRunner_closed2/Water Contact FR3/Subsystem1 ==
  F_drag : Inport
  angle : Inport  Port=2
  Mux : Mux  Inputs=2
  fcosq : Fcn  Expr=u(1)*cos(u(2))
  fsinq : Fcn  Expr=u(1)*sin(u(2))
  Fy : Outport
  Fx : Outport  Port=2
  wires:
  angle/1 -> Mux/2
  fcosq/1 -> Fy/1
  F_drag/1 -> Mux/1
  Mux/1 -> fcosq/1, fsinq/1
  fsinq/1 -> Fx/1

== system WaterRunner_closed2/Water Contact FR4/Quat to Euler1 ==
  Q : Inport
  f1 : Fcn  Expr=atan2( 2*(u(1)*u(2) + u(3)*u(4)) , 1-2*(u(2)^2+u(3)^2) )
  f3 : Fcn  Expr=atan2( 2*(u(1)*u(4) + u(2)*u(3)) , 1-2*(u(3)^2+u(4)^2) )
  phi_z : Outport
  phi_x : Outport  Port=2
  wires:
  Q/1 -> f1/1, f3/1
  f3/1 -> phi_z/1
  f1/1 -> phi_x/1

== system WaterRunner_closed2/Water Contact FR4/Subsystem ==
  y_c : Inport
  angle : Inport  Port=2
  v_n : Inport  Port=3
  ang_vel : Inport  Port=4
  Switch : Switch
  Switch1 : Switch
  water_model : Subsystem  mask{Cd=0.703, density=1000, y_w=water_level, R=0.02, g=-9.81}
      mask prompts: Cd "Drag Coefficient"; y_w "Water level"; R "Foot Radius"; g "Gravity constant (use negative)"
  water_model1 : Subsystem  mask{Cd=0.703, density=1000, y_w=water_level, R=0.005, g=-9.81}
      mask prompts: Cd "Drag Coefficient"; y_w "Water level"; R "Foot Radius"; g "Gravity constant (use negative)"
  Fk_w : Outport
  Fb_w : Outport  Port=2
  wires:
  angle/1 -> water_model1/2(angle), water_model/2(angle)
  ang_vel/1 -> water_model1/4(ang_vel), water_model/4(ang_vel)
  y_c/1 -> water_model1/1(y_c), water_model/1(y_c)
  v_n/1 -> water_model1/3(v_n), Switch/2, Switch1/2, water_model/3(v_n)
  water_model/1(Fk_w) -> Switch/1
  water_model/2(Fb_w) -> Switch1/1
  Switch/1 -> Fk_w/1
  water_model1/1(Fk_w) -> Switch/3
  water_model1/2(Fb_w) -> Switch1/3
  Switch1/1 -> Fb_w/1

== system WaterRunner_closed2/Water Contact FR4/Subsystem1 ==
  F_drag : Inport
  angle : Inport  Port=2
  Mux : Mux  Inputs=2
  fcosq : Fcn  Expr=u(1)*cos(u(2))
  fsinq : Fcn  Expr=u(1)*sin(u(2))
  Fy : Outport
  Fx : Outport  Port=2
  wires:
  angle/1 -> Mux/2
  fcosq/1 -> Fy/1
  F_drag/1 -> Mux/1
  Mux/1 -> fcosq/1, fsinq/1
  fsinq/1 -> Fx/1

== system WaterRunner_closed2/observer/averaging1 ==
  in : Inport
  Constant1 : Constant  Value=x_init
  Gain : Gain  Gain=1/T_win
  Integrator1 : Integrator
  Sum : Sum  Inputs=+-|
  Sum1 : Sum  Inputs=-+|
  Sum3 : Sum  Inputs=++|
  Transport Delay : TransportDelay  DelayTime=T_win
  out : Outport
  wires:
  in/1 -> Sum1/2
  Gain/1 -> Sum3/2
  Constant1/1 -> Sum3/1, Sum1/1
  Sum1/1 -> Integrator1/1
  Transport Delay/1 -> Sum/2
  Integrator1/1 -> Sum/1, Transport Delay/1
  Sum3/1 -> out/1
  Sum/1 -> Gain/1

== system WaterRunner_closed2/observer/averaging2 ==
  in : Inport
  Constant1 : Constant  Value=x_init
  Gain : Gain  Gain=1/T_win
  Integrator1 : Integrator
  Sum : Sum  Inputs=+-|
  Sum1 : Sum  Inputs=-+|
  Sum3 : Sum  Inputs=++|
  Transport Delay : TransportDelay  DelayTime=T_win
  out : Outport
  wires:
  in/1 -> Sum1/2
  Gain/1 -> Sum3/2
  Constant1/1 -> Sum3/1, Sum1/1
  Sum1/1 -> Integrator1/1
  Transport Delay/1 -> Sum/2
  Integrator1/1 -> Sum/1, Transport Delay/1
  Sum3/1 -> out/1
  Sum/1 -> Gain/1

== system WaterRunner_closed2/observer/averaging3 ==
  in : Inport
  Constant1 : Constant  Value=x_init
  Gain : Gain  Gain=1/T_win
  Integrator1 : Integrator
  Sum : Sum  Inputs=+-|
  Sum1 : Sum  Inputs=-+|
  Sum3 : Sum  Inputs=++|
  Transport Delay : TransportDelay  DelayTime=T_win
  out : Outport
  wires:
  in/1 -> Sum1/2
  Gain/1 -> Sum3/2
  Constant1/1 -> Sum3/1, Sum1/1
  Sum1/1 -> Integrator1/1
  Transport Delay/1 -> Sum/2
  Integrator1/1 -> Sum/1, Transport Delay/1
  Sum3/1 -> out/1
  Sum/1 -> Gain/1

== system WaterRunner_closed2/observer/averaging5 ==
  in : Inport
  Constant1 : Constant  Value=x_init
  Gain : Gain  Gain=1/T_win
  Integrator1 : Integrator
  Sum : Sum  Inputs=+-|
  Sum1 : Sum  Inputs=-+|
  Sum3 : Sum  Inputs=++|
  Transport Delay : TransportDelay  DelayTime=T_win
  out : Outport
  wires:
  in/1 -> Sum1/2
  Gain/1 -> Sum3/2
  Constant1/1 -> Sum3/1, Sum1/1
  Sum1/1 -> Integrator1/1
  Transport Delay/1 -> Sum/2
  Integrator1/1 -> Sum/1, Transport Delay/1
  Sum3/1 -> out/1
  Sum/1 -> Gain/1

== system WaterRunner_closed2/CPG_Network/split FL/enable ==
  in : Inport
  Constant1 : Constant
  Constant2 : Constant
  Fcn : Fcn  Expr=cos(u(1))
  Gain : Gain  Gain=.5
  Gain1 : Gain  Gain=.5
  Sign : Signum
  Sum1 : Sum  Inputs=|++
  Sum2 : Sum  Inputs=|-+
  pos : Outport
  neg : Outport  Port=2
  wires:
  Fcn/1 -> Sign/1
  Constant1/1 -> Sum1/2
  Sign/1 -> Sum2/1, Sum1/1
  Gain/1 -> pos/1
  in/1 -> Fcn/1
  Sum1/1 -> Gain/1
  Constant2/1 -> Sum2/2
  Gain1/1 -> neg/1
  Sum2/1 -> Gain1/1

== system WaterRunner_closed2/CPG_Network/split FL1/enable ==
  in : Inport
  Constant1 : Constant
  Constant2 : Constant
  Fcn : Fcn  Expr=cos(u(1))
  Gain : Gain  Gain=.5
  Gain1 : Gain  Gain=.5
  Sign : Signum
  Sum1 : Sum  Inputs=|++
  Sum2 : Sum  Inputs=|-+
  pos : Outport
  neg : Outport  Port=2
  wires:
  Fcn/1 -> Sign/1
  Constant1/1 -> Sum1/2
  Sign/1 -> Sum2/1, Sum1/1
  Gain/1 -> pos/1
  in/1 -> Fcn/1
  Sum1/1 -> Gain/1
  Constant2/1 -> Sum2/2
  Gain1/1 -> neg/1
  Sum2/1 -> Gain1/1

== system WaterRunner_closed2/CPG_Network/split FL2/enable ==
  in : Inport
  Constant1 : Constant
  Constant2 : Constant
  Fcn : Fcn  Expr=cos(u(1))
  Gain : Gain  Gain=.5
  Gain1 : Gain  Gain=.5
  Sign : Signum
  Sum1 : Sum  Inputs=|++
  Sum2 : Sum  Inputs=|-+
  pos : Outport
  neg : Outport  Port=2
  wires:
  Sum2/1 -> Gain1/1
  Gain1/1 -> neg/1
  Constant2/1 -> Sum2/2
  Sum1/1 -> Gain/1
  in/1 -> Fcn/1
  Gain/1 -> pos/1
  Sign/1 -> Sum1/1, Sum2/1
  Constant1/1 -> Sum1/2
  Fcn/1 -> Sign/1

== system WaterRunner_closed2/CPG_Network/split FL3/enable ==
  in : Inport
  Constant1 : Constant
  Constant2 : Constant
  Fcn : Fcn  Expr=cos(u(1))
  Gain : Gain  Gain=.5
  Gain1 : Gain  Gain=.5
  Sign : Signum
  Sum1 : Sum  Inputs=|++
  Sum2 : Sum  Inputs=|-+
  pos : Outport
  neg : Outport  Port=2
  wires:
  Fcn/1 -> Sign/1
  Constant1/1 -> Sum1/2
  Sign/1 -> Sum2/1, Sum1/1
  Gain/1 -> pos/1
  in/1 -> Fcn/1
  Sum1/1 -> Gain/1
  Constant2/1 -> Sum2/2
  Gain1/1 -> neg/1
  Sum2/1 -> Gain1/1

== system WaterRunner_closed2/Tail/Water Contact HR1/water_model ==
  y_c : Inport
  angle : Inport  Port=2
  v_n : Inport  Port=3
  ang_vel : Inport  Port=4
  Gain1 : Gain  Gain=Cd*density
  Gain3 : Gain  Gain=-1
  Product1 : Product  RndMeth=Zero
  Product2 : Product  RndMeth=Zero
  Subsystem : Subsystem
  Subsystem1 : Subsystem
  Subsystem2 : Subsystem
  Subsystem3 : Subsystem
  Sum : Sum  Inputs=|++
  Sum2 : Sum  Inputs=-+|
  damper_force1 : Subsystem
  damper_force2 : Subsystem
  Fb_w : Outport
  wires:
  Gain1/1 -> Gain3/1
  Sum/1 -> Gain1/1
  Product2/1 -> Sum/2
  ang_vel/1 -> damper_force1/2(a), damper_force2/2(a), Subsystem3/2(dtheta), Subsystem2/1(dtheta)
  v_n/1 -> damper_force1/3(b), damper_force2/3(b), Subsystem3/1(vel), Subsystem2/2(v)
  angle/1 -> Subsystem/2(angle)
  y_c/1 -> Subsystem/1(y_c)
  Product1/1 -> Sum/1
  damper_force2/1(Int_b) -> Product1/1
  damper_force1/1(Int_b) -> Product2/1
  Subsystem2/1(S+) -> Sum2/1, Product1/2
  Subsystem2/2(S-) -> Sum2/2
  Sum2/1 -> Product2/2
  Subsystem3/1(mid_b) -> Subsystem2/3(r0), Subsystem1/2(r0)
  Gain3/1 -> Fb_w/1
  Subsystem/1(up_b) -> damper_force2/1(up_b), Subsystem1/1(r)
  Subsystem1/1(r00) -> damper_force1/1(up_b)

== system WaterRunner_closed2/Water Contact FR1/Subsystem/water_model ==
  y_c : Inport
  angle : Inport  Port=2
  v_n : Inport  Port=3
  ang_vel : Inport  Port=4
  Gain : Gain
  Gain1 : Gain  Gain=Cd*density
  Gain2 : Gain  Gain=Cd*density
  Gain3 : Gain  Gain=-1
  Product1 : Product  RndMeth=Zero
  Product2 : Product  RndMeth=Zero
  Subsystem : Subsystem
  Subsystem1 : Subsystem
  Subsystem2 : Subsystem
  Subsystem3 : Subsystem
  Subsystem4 : Subsystem
  Sum : Sum  Inputs=|++
  Sum2 : Sum  Inputs=-+|
  damper_force1 : Subsystem
  damper_force2 : Subsystem
  spring_force : Subsystem
  Fk_w : Outport
  Fb_w : Outport  Port=2
  wires:
  Subsystem4/1(r00) -> damper_force1/1(up_b)
  Subsystem3/1(mid_b) -> Subsystem4/2(r0), Subsystem2/3(r0)
  Gain1/1 -> Gain3/1
  Sum/1 -> Gain1/1
  Product2/1 -> Sum/2
  Subsystem1/2(b) -> spring_force/3(b)
  spring_force/1(Int_k) -> Gain2/1
  Gain2/1 -> Gain/1
  ang_vel/1 -> damper_force1/2(a), damper_force2/2(a), Subsystem3/2(dtheta), Subsystem2/1(dtheta)
  v_n/1 -> damper_force1/3(b), damper_force2/3(b), Subsystem3/1(vel), Subsystem2/2(v)
  Subsystem1/1(a) -> spring_force/2(a)
  angle/1 -> Subsystem/2(angle), Subsystem1/2(angle)
  y_c/1 -> Subsystem/1(y_c), Subsystem1/1(y_c)
  Subsystem/1(up_b) -> damper_force2/1(up_b), Subsystem4/1(r), spring_force/1(up_b)
  Product1/1 -> Sum/1
  damper_force2/1(Int_b) -> Product1/1
  damper_force1/1(Int_b) -> Product2/1
  Subsystem2/1(S+) -> Sum2/1, Product1/2
  Subsystem2/2(S-) -> Sum2/2
  Sum2/1 -> Product2/2
  Gain/1 -> Fk_w/1
  Gain3/1 -> Fb_w/1

== system WaterRunner_closed2/Water Contact FR1/Subsystem/water_model1 ==
  y_c : Inport
  angle : Inport  Port=2
  v_n : Inport  Port=3
  ang_vel : Inport  Port=4
  Gain : Gain
  Gain1 : Gain  Gain=Cd*density
  Gain2 : Gain  Gain=Cd*density
  Gain3 : Gain  Gain=-1
  Product1 : Product  RndMeth=Zero
  Product2 : Product  RndMeth=Zero
  Subsystem : Subsystem
  Subsystem1 : Subsystem
  Subsystem2 : Subsystem
  Subsystem3 : Subsystem
  Subsystem4 : Subsystem
  Sum : Sum  Inputs=|++
  Sum2 : Sum  Inputs=-+|
  damper_force1 : Subsystem
  damper_force2 : Subsystem
  spring_force : Subsystem
  Fk_w : Outport
  Fb_w : Outport  Port=2
  wires:
  Subsystem4/1(r00) -> damper_force1/1(up_b), Subsystem2/3(r0)
  Subsystem3/1(mid_b) -> Subsystem4/2(r0)
  Gain1/1 -> Gain3/1
  Sum/1 -> Gain1/1
  Product2/1 -> Sum/2
  Subsystem1/2(b) -> spring_force/3(b)
  spring_force/1(Int_k) -> Gain2/1
  Gain2/1 -> Gain/1
  ang_vel/1 -> damper_force1/2(a), damper_force2/2(a), Subsystem3/2(dtheta), Subsystem2/1(dtheta)
  v_n/1 -> damper_force1/3(b), damper_force2/3(b), Subsystem3/1(vel), Subsystem2/2(v)
  Subsystem1/1(a) -> spring_force/2(a)
  angle/1 -> Subsystem/2(angle), Subsystem1/2(angle)
  y_c/1 -> Subsystem/1(y_c), Subsystem1/1(y_c)
  Subsystem/1(up_b) -> damper_force2/1(up_b), Subsystem4/1(r), spring_force/1(up_b)
  Product1/1 -> Sum/1
  damper_force2/1(Int_b) -> Product1/1
  damper_force1/1(Int_b) -> Product2/1
  Subsystem2/1(S+) -> Sum2/1, Product1/2
  Subsystem2/2(S-) -> Sum2/2
  Sum2/1 -> Product2/2
  Gain/1 -> Fk_w/1
  Gain3/1 -> Fb_w/1
